simulink model "LUPA"  (R2025b)
settings: Solver=FixedStepAuto  StartTime=0.0  StopTime=inf  FixedStep=Ts  RelTol=1e-3
PreLoadFcn:
  | addpath(genpath('utils'))
model workspace (MAT data in the model file):
  Sig = Simulink.Signal
  Sig.Dimensions = -1
  Sig.DimensionsMode = 'auto'
  Sig.Complexity = 'auto'
  Sig.SampleTime = -1
  Sig.SamplingMode = 'auto'
  Sig.DataType = 'auto'
values from neighbouring files (symbols this model uses):
  C = 258.803991051052    (= 258.803991051)    [AOE_constants.m]
  CL = 13    [initLUPA.m]
  ExcelGains = table2array(ExcelGains)    [initLUPA.m]
  gainTstep = wavePeriod*10    (= 22.5)    [initLUPA.m]
  Kt = 7.86    [initLUPA.m]
  rampTime = 20    [initLUPA.m]
  sprocketPitchRadius = 0.101854    [initLUPA.m]
  Ts = 0.001    [initLUPA.m]
undefined symbols (not defined in the file or in its folder): AOE, DiscIntNeverNeededParam, drawWire_m, drawWire_mpers, eCATstate, linearPower_W, netForce_N, opState, pos_filt_rad, tet, vel_filt_radpers
libraries: slrealtimeethercatlib x16, slrealtimeloglib x10, simulink x7, dspfdesign x6, eeGeneralControl x3, slrealtimeutilitieslib x2, dspstat3 x2, slrealtimeptplib x1, slrealtimetgmanagement x1
(part 1 of 2)
settings Model: SimulationMode=external  ExtModeEnableFloating=off  Creator=HWRL user  LastModifiedBy=Wave User
settings SolverCC: ConcurrentTasks=on  PositivePriorityOrder=on
settings DataIOCC: ExternalInput=ds  LoadExternalInput=on
settings OptimizationCC: BlockReduction=off  OptimizeBlockIOStorage=off  ReuseModelBlockBuffer=off
settings DebuggingCC: TasksWithSamePriorityMsg=none  ParameterOverflowMsg=warning  ParameterPrecisionLossMsg=none  UnconnectedInputMsg=warning  UnconnectedOutputMsg=warning  UnconnectedLineMsg=warning
settings HardwareCC: ProdBitPerLong=64.0  ProdLongLongMode=on  ProdHWDeviceType=Intel->x86-64 (Linux 64)
settings ModelReferenceCC: EnableRefExpFcnMdlSchedulingChecks=on
settings SFSimCC: SimTargetLang=C++  SimDLTargetLibrary=mkl-dnn
settings RTWCC: SystemTargetFile=speedgoat.tlc  TemplateMakefile=slrealtime_default_tmf  RTWVerbose=off  Toolchain=Simulink Real-Time Toolchain  BuildConfiguration=Faster Runs  CodeExecutionProfiling=on  TargetLang=C++  GPUComputeCapability=3.5  DLArmComputeVersion=19.05  Description=Speedgoat Real-Time Target Machine
settings SimulinkRealTimeTargetCC: SLRTFileLogMaxRuns=1.0  ExtModeMaxTrigDuration=10.0  ExtModeStaticAllocSize=1000000.0  ExtModeTransport=0.0  MultiwordLength=2048.0  DynamicStringBufferSize=256.0  PreserveMATLABNamespacesInGeneratedCode=on  SubcomponentCodeInterfacePackaging=Reusable function  InstructionSetFMA=off  LogToMDFFile=off

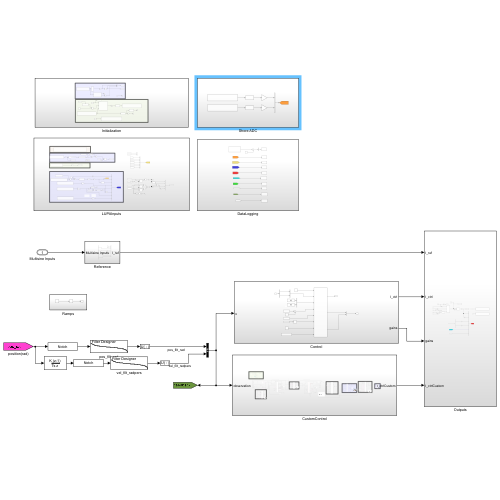
[thumbnail: Simulink's stored preview of the top-level diagram]
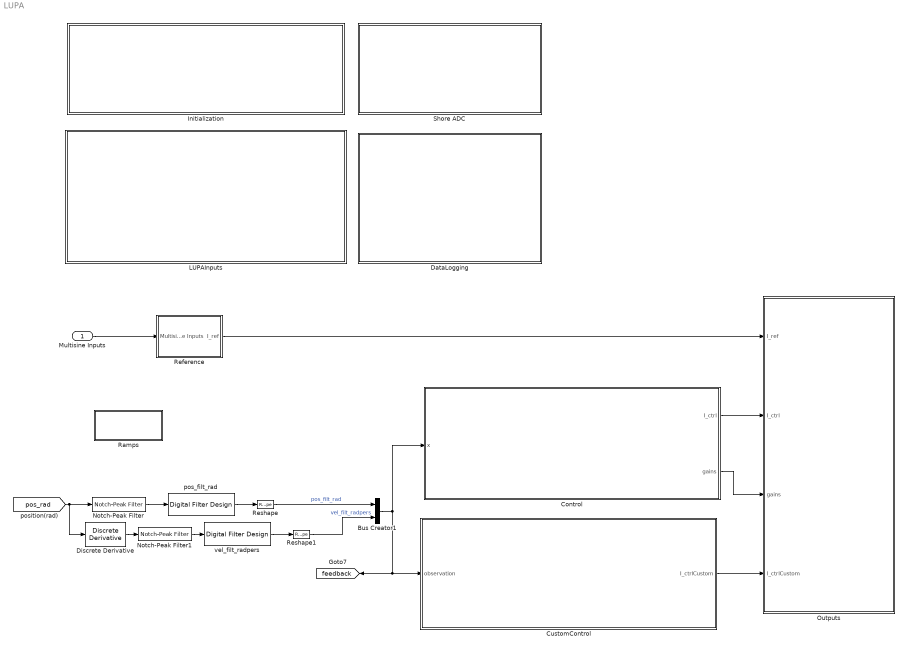
== system LUPA ==
  Multisine Inputs : Inport  OutDataTypeStr=Bus: refSigs
  Bus Creator1 : BusCreator  Inputs=pos_filt_rad,vel_filt_radpers
  Control : Subsystem
  CustomControl : Subsystem
  DataLogging : Subsystem
  Discrete Derivative : simulink/Discrete/Discrete Derivative  gainval=1.0  ICPrevScaledInput=0.0  OutMin=[]  OutMax=[]  OutDataType=fixdt(1, 16)  OutScaling=2^-10  DoSatur=off
  Initialization : Subsystem
  LUPAInputs : Subsystem
  Notch-Peak Filter : dspfdesign/Notch-Peak Filter  Specification=Bandwidth and center frequency  BandwidthPort=off  Bandwidth=10  QualityFactorPort=off  QualityFactor=5  CenterFrequencyPort=off  CenterFrequency=50  BandwidthCoefficientPort=off  BandwidthCoefficient=0.72654  CenterFrequencyCoefficientPort=off  CenterFrequencyCoefficient=0  Output=Notch  SampleRateMode=Specify on dialog  SampleRate=1000  SimulateUsing=Code generation
  Notch-Peak Filter1 : dspfdesign/Notch-Peak Filter  Specification=Bandwidth and center frequency  BandwidthPort=off  Bandwidth=10  QualityFactorPort=off  QualityFactor=5  CenterFrequencyPort=off  CenterFrequency=50  BandwidthCoefficientPort=off  BandwidthCoefficient=0.72654  CenterFrequencyCoefficientPort=off  CenterFrequencyCoefficient=0  Output=Notch  SampleRateMode=Specify on dialog  SampleRate=1000  SimulateUsing=Code generation
  Outputs : Subsystem
  Ramps : Subsystem
  Reference : Subsystem
  Reshape : Reshape
  Reshape1 : Reshape
  Shore ADC : Subsystem
  pos_filt_rad : dspfdesign/Digital Filter Design  mwdsp_browser_bugfix_var=off
  vel_filt_radpers : dspfdesign/Digital Filter Design  mwdsp_browser_bugfix_var=off
  tag scope: feedback=global
  wires:
  Control/1(I_ctrl) -> Outputs/2(I_ctrl)
  Bus Creator1/1 -> Control/1(x), CustomControl/1(observation), [feedback]
  [pos_rad] -> Discrete Derivative/1, Notch-Peak Filter/1
  Control/2(gains) -> Outputs/3(gains)
  CustomControl/1(I_ctrlCustom) -> Outputs/4(I_ctrlCustom)
  Reference/1(I_ref) -> Outputs/1(I_ref)
  Multisine Inputs/1 -> Reference/1(Multisine Inputs)
  Notch-Peak Filter/1 -> pos_filt_rad/1
  Notch-Peak Filter1/1 -> vel_filt_radpers/1
  Discrete Derivative/1 -> Notch-Peak Filter1/1
  pos_filt_rad/1 -> Reshape/1
  vel_filt_radpers/1 -> Reshape1/1
  Reshape/1 -> Bus Creator1/1  "pos_filt_rad"
  Reshape1/1 -> Bus Creator1/2  "vel_filt_radpers"

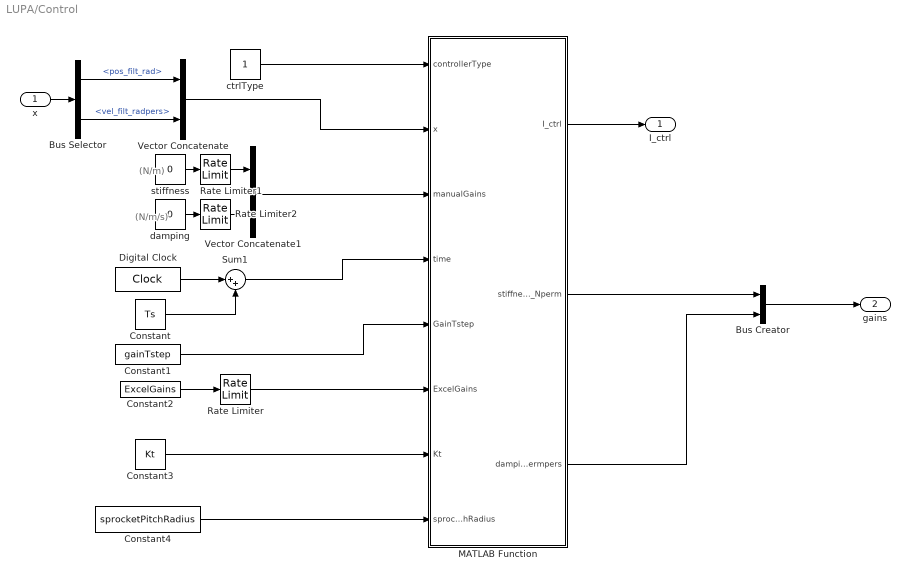
== system LUPA/Control ==
  note: (N/m/s)
  note: (N/m)
  x : Inport
  Bus Creator : BusCreator  Inputs=2
  Bus Selector : BusSelector  OutputSignals=pos_filt_rad,vel_filt_radpers
  Constant : Constant  Value=Ts
  Constant1 : Constant  Value=gainTstep
  Constant2 : Constant  Value=ExcelGains  VectorParams1D=off
  Constant3 : Constant  Value=Kt
  Constant4 : Constant  Value=sprocketPitchRadius
  Digital Clock : DigitalClock  SampleTime=Ts
  MATLAB Function : MATLAB Function  TreatAsAtomicUnit=on
  Rate Limiter : RateLimiter  RisingSlewLimit=200  FallingSlewLimit=-200  SampleTimeMode=inherited
  Rate Limiter1 : RateLimiter  RisingSlewLimit=200  FallingSlewLimit=-200  SampleTimeMode=inherited
  Rate Limiter2 : RateLimiter  RisingSlewLimit=200  FallingSlewLimit=-200  SampleTimeMode=inherited
  Sum1 : Sum  Inputs=|++
  Vector Concatenate : Concatenate  Mode=Multidimensional array
  Vector Concatenate1 : Concatenate  Mode=Multidimensional array
  ctrlType : Constant
  damping : Constant  Value=0
  stiffness : Constant  Value=0
  I_ctrl : Outport
  gains : Outport  Port=2
  wires:
  stiffness/1 -> Rate Limiter1/1
  Constant1/1 -> MATLAB Function/5(GainTstep)
  Constant/1 -> Sum1/2
  Vector Concatenate1/1 -> MATLAB Function/3(manualGains)
  Digital Clock/1 -> Sum1/1
  x/1 -> Bus Selector/1
  Sum1/1 -> MATLAB Function/4(time)
  Constant4/1 -> MATLAB Function/8(sprocketPitchRadius)
  damping/1 -> Rate Limiter2/1
  Vector Concatenate/1 -> MATLAB Function/2(x)
  ctrlType/1 -> MATLAB Function/1(controllerType)
  Constant3/1 -> MATLAB Function/7(Kt)
  Constant2/1 -> Rate Limiter/1
  Bus Selector/1 -> Vector Concatenate/1  "<pos_filt_rad>"
  Bus Selector/2 -> Vector Concatenate/2  "<vel_filt_radpers>"
  MATLAB Function/1(I_ctrl) -> I_ctrl/1
  MATLAB Function/2(stiffness_Nperm) -> Bus Creator/1
  MATLAB Function/3(damping_Npermpers) -> Bus Creator/2
  Bus Creator/1 -> gains/1
  Rate Limiter/1 -> MATLAB Function/6(ExcelGains)
  Rate Limiter1/1 -> Vector Concatenate1/1
  Rate Limiter2/1 -> Vector Concatenate1/2

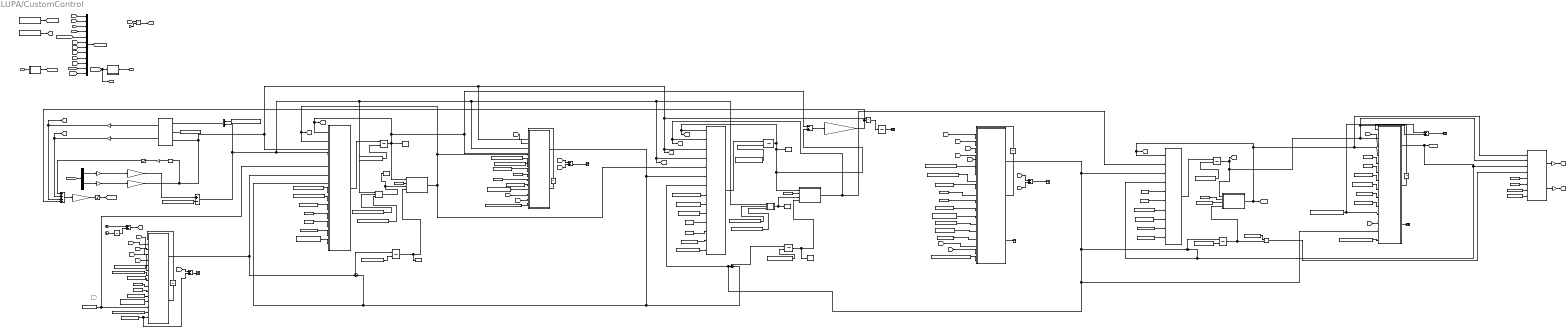
== system LUPA/CustomControl ==
  note: HWRL Code
  note: Outlet Piston Chamber 1 Valve
  note: Useful Power
  note: Outlet Tank Valve
  note: Outlet Piston Valve
  note: Inlet Piston valve
  observation : Inport
  Add1 : Sum  Inputs=+-
  Add{2..3,7,9} (4 alike) : Sum  Inputs=-+
  Add8 : Sum  Inputs=++++  RndMeth=Simplest
  Assertion : Assertion  AssertionFailFcn=Ch1C1 mass is zero
  Assertion1 : Assertion  AssertionFailFcn=Ch1C1 pressure is zero
  Assertion2 : Assertion  AssertionFailFcn=Ch2C1 pressure is zero  StopWhenAssertionFail=off
  Assertion3 : Assertion  AssertionFailFcn=Ch2C1 mass is zero  StopWhenAssertionFail=off
  Assertion4 : Assertion  AssertionFailFcn=Ch1C1 volume is zero
  Assertion5 : Assertion  AssertionFailFcn=Ch2C1 volume is zero  StopWhenAssertionFail=off
  Atmospheric pressure2 : Constant  Value=AOE.AtmPressure
  Atmospheric temperature : Constant  Value=AOE.AtmTemperature
  Bus Selector1 : BusSelector  OutputSignals=pos_filt_m,vel_filt_mpers
  Clock : Clock
  Clock1 : Clock
  Constant : Constant  Value=sprocketPitchRadius
  Constant1 : Constant  Value=Kt
  Constant{4..6,10,22,27,30,35,39,43,61} (11 alike) : Constant  Value=AOE.Rs
  Constant11 : Constant  Value=AOE.Cp
  Constant12 : Constant  Value=AOE.Chamber1.InitialAirMass
  Constant{2,14,24,37,56} (5 alike) : Constant  Value=AOE.Cylinder.HeatConvection
  Constant16 : Constant  Value=AOE.Chamber2.InitialPistonPosition
  Constant17 : Constant  Value=AOE.Cylinder.Diameter
  Constant18 : Constant  Value=AOE.Chamber2.InitialAirMass
  Constant19 : Constant  Value=AOE.Chamber1.InitialPressure
  Constant20 : Constant  Value=AOE.Chamber2.InitialPressure
  Constant21 : Constant  Value=AOE.OutletTankOrifice.CrossSectionalArea
  Constant{7,23,28,31,40,47,62} (7 alike) : Constant  Value=AOE.gma
  Constant25 : Constant  Value=AOE.Tank.InitialAirMass
  Constant{9,26,38,42,52,57,64} (7 alike) : Constant  Value=AOE.WaterTemperature
  Constant{8,29,41,46,49,51,63} (7 alike) : Constant  Value=AOE.Cylinder.CrossSectionalArea
  Constant{3,48,50,55,60} (5 alike) : Constant  Value=AOE.Tank.Volume
  Constant32 : Constant  Value=AOE.Tank.HeatConvection
  Constant33 : Constant  Value=AOE.Tank.InitialPressure
  Constant34 : Constant  Value=AOE.Tank.SurfaceArea
  Constant44 : Constant  Value=AOE.Chamber2.InitialPistonPosition
  Constant53 : Constant  Value=AOE.Tank.HeatConvection
  Constant54 : Constant  Value=AOE.Tank.SurfaceArea
  Constant58 : Constant  Value=AOE.Tank.HeatConvection
  Constant59 : Constant  Value=AOE.Tank.SurfaceArea
  Constant65 : Constant  Value=AOE.InletCylinderOrifice.CrossSectionalArea
  Constant66 : Constant  Value=AOE.OutletCylinderOrifice.CrossSectionalArea
  Constant67 : Constant  Value=AOE.Chamber1Chamber2Orifice.CrossSectionalArea
  Coulomb & Viscous Friction Unit1 : simulink/Discontinuities/Coulomb & Viscous Friction  offset=0  gain=AOE.Cylinder.CoulombFrictionGain
  CustomControl : BusCreator  Inputs=12
  Cyl D{,1..3} (4 alike) : Constant  Value=AOE.Cylinder.Diameter
  Determining Useful Energy : MATLAB Function
      settings: MinAlgLoopOccurrences=on
  Discrete-Time Integrator : DiscreteIntegrator  InitialConditionSource=external  InitialCondition=101.3  SampleTime=-1  LimitOutput=on  LowerSaturationLimit=0  ICPrevOutput=DiscIntNeverNeededParam  ICPrevScaledInput=DiscIntNeverNeededParam
  Discrete-Time Integrator10 : DiscreteIntegrator  InitialConditionSource=external  InitialCondition=1.2754*(10)*.25*pi*0.5^2  SampleTime=-1  LimitOutput=on  LowerSaturationLimit=0  ICPrevOutput=DiscIntNeverNeededParam  ICPrevScaledInput=DiscIntNeverNeededParam
  Discrete-Time Integrator11 : DiscreteIntegrator  InitialConditionSource=external  InitialCondition=1.2754*(2+.05)*.25*pi*2.14^2  SampleTime=-1  LimitOutput=on  LowerSaturationLimit=0  ICPrevOutput=DiscIntNeverNeededParam  ICPrevScaledInput=DiscIntNeverNeededParam
  Discrete-Time Integrator12 : DiscreteIntegrator  InitialConditionSource=external  InitialCondition=101.3  SampleTime=-1  LimitOutput=on  LowerSaturationLimit=0  ICPrevOutput=DiscIntNeverNeededParam  ICPrevScaledInput=DiscIntNeverNeededParam
  Discrete-Time Integrator2 : DiscreteIntegrator  InitialConditionSource=external  InitialCondition=1.2754*(2+.05)*.25*pi*2.14^2  SampleTime=-1  LimitOutput=on  LowerSaturationLimit=0  ICPrevOutput=DiscIntNeverNeededParam  ICPrevScaledInput=DiscIntNeverNeededParam
  Endstop Forces Unit1 : Subsystem
  Energy : DiscreteIntegrator  SampleTime=-1  LimitOutput=on  ICPrevOutput=DiscIntNeverNeededParam  ICPrevScaledInput=DiscIntNeverNeededParam
  Exergy : Gain
  Fh : Gain  OutDataTypeStr=double
  Fl : Gain  OutDataTypeStr=double
  Force : Gain  Gain=AOE.lambda^-3
  Force Limit : Saturate  UpperLimit=500  LowerLimit=-500
  ForceToCurrent : Subsystem
  From1 : From  Commented=on  GotoTag=TC1
  Gain : Gain  Gain=-1
  Gain1 : Gain  Gain=AOE.Cylinder.CrossSectionalArea
  Gain2 : Gain  Gain=AOE.lambda
  Gain3 : Gain  Gain=AOE.lambda^0.5
  P_pto : Product
  Power : Gain
  Pressure Chamber1 Box Unit1 : MATLAB Function
      settings: MinAlgLoopOccurrences=on
  Pressure Chamber2 Box Unit1 : MATLAB Function
  Pressure Tank Box Unit1 : MATLAB Function
      settings: MinAlgLoopOccurrences=on
  Pressure into Chamber 1 : Constant  Value=AOE.Chamber1.PressureIn
  Product2 : Product
  Product3 : Product  Inputs=/*
  Revised Cylinder Outlet Valve Model : MATLAB Function
      settings: MinAlgLoopOccurrences=on
  Revised Valve Model Chamber1Chamber2 Unit1 : MATLAB Function
      settings: MinAlgLoopOccurrences=on
  Revised Valve Model Inlet Unit1 : MATLAB Function
      settings: MinAlgLoopOccurrences=on
  Revised Valve Tank Outlet : MATLAB Function
      settings: MinAlgLoopOccurrences=on
  RotaryToLinear : Subsystem
  Saturation : Saturate  UpperLimit=AOE.Cylinder.CoulombFrictionLimit  LowerLimit=-AOE.Cylinder.CoulombFrictionLimit
  Sum : Sum  Inputs=+-
  Sum1 : Sum  Inputs=-+
  Sum2 : Sum  Inputs=-+
  Sum3 : Sum  Inputs=+|-
  Sum6 : Sum
  Temperature Chamber1 Box Unit1 : MATLAB Function
      settings: MinAlgLoopOccurrences=on
  Temperature Chamber2 Box Unit1 : MATLAB Function
      settings: MinAlgLoopOccurrences=on
  Temperature Tank Box Unit1 : MATLAB Function
  Terminator{,1..3,5..7} (7 alike) : Terminator
  Unit Delay{,1..4} (5 alike) : UnitDelay  SampleTime=-1
  Volume Chamber1 Box Unit1 : MATLAB Function
      settings: MinAlgLoopOccurrences=on
  Volume Chamber2 Box Unit1 : MATLAB Function
      settings: MinAlgLoopOccurrences=on
  cylinder equilibrium offset position{1,3..5} (4 alike) : Constant  Value=AOE.Chamber1.InitialPistonPosition
  cylinder equilibrium offset position2 : Constant  Value=AOE.Chamber2.InitialPistonPosition
  cylinder equilibrium offset position6 : Constant  Value=AOE.Chamber2.InitialPistonPosition
  cylinder initial offset : Constant  Value=AOE.Cylinder.InitialOffset
  cylinder total Length : Constant  Value=AOE.Cylinder.Length
  override2 : Constant  Value=AOE.OutletTankOrifice.CrackPressure
  pos_m : Gain
  tankPressure : DiscreteIntegrator  InitialConditionSource=external  InitialCondition=101.3  SampleTime=-1  LimitOutput=on  LowerSaturationLimit=0  ICPrevOutput=DiscIntNeverNeededParam  ICPrevScaledInput=DiscIntNeverNeededParam
  tempAmb2 : Constant  Value=AOE.AtmTemperature
  vel_mpers : Gain
  z_off : Sum  Inputs=+-  RndMeth=Simplest
  I_ctrlCustom : Outport
  tag scope: CustomControl=global, Kt=global, P_PTO=global, sprocketPitchRadius=global
  wires:
  Constant/1 -> [sprocketPitchRadius]
  Constant1/1 -> [Kt]
  ForceToCurrent/1(Out1) -> I_ctrlCustom/1
  [F_PTO] -> P_pto/1
  [v] -> P_pto/2
  P_pto/1 -> [P_PTO]  "P_PTO"
  observation/1 -> RotaryToLinear/1(rotational)
  CustomControl/1 -> [CustomControl]
  [F_PTO] -> CustomControl/1  "F_PTO"
  [z] -> CustomControl/2  "z"
  [v] -> CustomControl/3  "v"
  [P_PTO] -> CustomControl/4  "P_PTO"
  [EnableCustControl] -> CustomControl/5  "customControlEnable"
  Clock/1 -> Add1/1
  Volume Chamber2 Box Unit1/1(V) -> Assertion5/1, Temperature Chamber2 Box Unit1/3(V)  "Chamber2 volume"
  Revised Cylinder Outlet Valve Model/2(mdotMax) -> Unit Delay2/1
  Constant2/1 -> Revised Valve Model Chamber1Chamber2 Unit1/13(hC)
  Pressure into Chamber 1/1 -> Add9/2, Revised Valve Model Inlet Unit1/16(Pin)
  Endstop Forces Unit1/1(F_stop_hi) -> Fl/1  "Fstop_high"
  Atmospheric pressure2/1 -> Determining Useful Energy/8(Pamb)
  Discrete-Time Integrator11/1 -> Temperature Chamber1 Box Unit1/4(m), Assertion/1  "chamber1 air mass"
  Volume Chamber1 Box Unit1/1(V) -> Assertion4/1, Temperature Chamber1 Box Unit1/3(V)  "Chamber1 Volume"
  [response] -> Bus Selector1/1
  Cyl D3/1 -> Revised Valve Model Chamber1Chamber2 Unit1/9(DC)
  [PC1] -> Add9/1
  cylinder equilibrium offset position6/1 -> Revised Cylinder Outlet Valve Model/7(LC)
  tankPressure/1 -> [PT], Temperature Tank Box Unit1/1(P), Revised Valve Tank Outlet/3(PT), Determining Useful Energy/2(P), Add3/2  "Tank pressure"
  Unit Delay4/1 -> Revised Valve Model Inlet Unit1/1(mdotMaxOld)
  Constant56/1 -> Revised Valve Model Inlet Unit1/13(hC)
  Constant28/1 -> Pressure Chamber2 Box Unit1/12(gma)
  Constant32/1 -> Pressure Tank Box Unit1/7(h)
  [xDot] -> Revised Valve Model Inlet Unit1/5(xdot)
  override2/1 -> Add3/1, Revised Valve Tank Outlet/11(Pcrack)
  [TC1] -> Revised Valve Model Inlet Unit1/4(TC1)
  Constant4/1 -> Temperature Chamber1 Box Unit1/2(Rs)
  [TimeStep] -> Revised Cylinder Outlet Valve Model/2(TimeStep)
  Unit Delay1/1 -> Add1/2
  Constant39/1 -> Revised Valve Model Chamber1Chamber2 Unit1/10(Rs)
  [PC1] -> Add7/2
  Constant8/1 -> Pressure Chamber1 Box Unit1/9(A)
  Sum2/1 -> Discrete-Time Integrator2/1
  Constant57/1 -> Revised Valve Tank Outlet/7(Tw)
  Revised Valve Tank Outlet/3(beta) -> Terminator5/1
  Discrete-Time Integrator10/1 -> Product3/2, Temperature Tank Box Unit1/4(m)  "Tank air mas"
  Constant60/1 -> Revised Valve Tank Outlet/9(VT)
  Constant35/1 -> Temperature Tank Box Unit1/2(Rs)
  Gain1/1 -> Add8/4, Product2/2  "Pressure Potential Force"
  [TC2] -> Revised Valve Model Chamber1Chamber2 Unit1/15(TC2)
  Cyl D1/1 -> Revised Cylinder Outlet Valve Model/9(DC)
  Constant61/1 -> Revised Valve Model Inlet Unit1/10(Rs)
  Product3/1 -> Determining Useful Energy/4(Density)
  Constant12/1 -> Discrete-Time Integrator11/2
  Constant66/1 -> Revised Cylinder Outlet Valve Model/19(A)
  Unit Delay2/1 -> Revised Cylinder Outlet Valve Model/1(mdotMaxOld)
  Revised Cylinder Outlet Valve Model/1(MassFlow) -> Revised Valve Tank Outlet/13(mDotIn), Pressure Chamber2 Box Unit1/7(mdot3), Sum2/1, Sum3/1, Pressure Tank Box Unit1/3(mdot1)  "Outlet cylinder"
  cylinder equilibrium offset position3/1 -> Revised Valve Model Chamber1Chamber2 Unit1/7(LC)
  Constant64/1 -> Revised Valve Model Inlet Unit1/12(Tw)
  Add8/1 -> Force/1  "Total Reaction Force"
  Constant27/1 -> Pressure Chamber2 Box Unit1/11(Rs)
  [TC2] -> Revised Valve Tank Outlet/12(TC)
  [TC2] -> Revised Cylinder Outlet Valve Model/4(TC)
  Constant6/1 -> Pressure Chamber1 Box Unit1/11(Rs)
  Constant62/1 -> Revised Valve Model Inlet Unit1/11(gma)
  Constant53/1 -> Revised Cylinder Outlet Valve Model/14(hT)
  Constant26/1 -> Pressure Chamber2 Box Unit1/13(Tw)
  Add1/1 -> [TimeStep]
  [PT] -> Revised Cylinder Outlet Valve Model/17(PT)
  Discrete-Time Integrator2/1 -> Temperature Chamber2 Box Unit1/4(m), Assertion3/1  "Chamber2 air mass"
  [TimeStep] -> Revised Valve Tank Outlet/2(TimeStep)
  Add2/1 -> Terminator2/1
  Coulomb & Viscous Friction Unit1/1 -> Gain/1
  Revised Valve Model Chamber1Chamber2 Unit1/2(mdotMax) -> Unit Delay3/1
  Unit Delay/1 -> Revised Valve Tank Outlet/1(mdotMaxOld)
  cylinder equilibrium offset position5/1 -> Revised Valve Model Inlet Unit1/7(LC)
  Sum6/1 -> Endstop Forces Unit1/1(x)  "Piston Position"
  Constant21/1 -> Revised Valve Tank Outlet/14(A)
  Constant44/1 -> Sum6/1
  Constant43/1 -> Revised Cylinder Outlet Valve Model/10(Rs)
  Pressure Chamber1 Box Unit1/1(Pdot) -> Discrete-Time Integrator/1  "pdot(t)"
  Gain2/1 -> z_off/1  "x"
  Constant63/1 -> Revised Valve Model Inlet Unit1/8(AC)
  Constant48/1 -> Temperature Tank Box Unit1/3(V)
  Add7/1 -> Terminator6/1
  Endstop Forces Unit1/2(F_stop_lo) -> Fh/1  "Fstop_high"
  Cyl D2/1 -> Revised Valve Model Inlet Unit1/9(DC)
  Gain3/1 -> Coulomb & Viscous Friction Unit1/1, Pressure Chamber1 Box Unit1/3(xdot), Revised Valve Model Chamber1Chamber2 Unit1/3(xdot), [xDot], Pressure Chamber2 Box Unit1/3(xdot), Product2/1, Endstop Forces Unit1/3(xdot(t))  "Xdot"
  Revised Valve Model Inlet Unit1/1(MassFlow) -> Sum/1, Pressure Chamber1 Box Unit1/6(mdot1)  "Inlet Cylinder MassFlow to Cyl"
  Constant17/1 -> Pressure Chamber2 Box Unit1/10(D)
  Constant58/1 -> Revised Valve Tank Outlet/8(hT)
  Constant65/1 -> Revised Valve Model Inlet Unit1/15(A)
  Determining Useful Energy/1(Exergy) -> Exergy/1
  Revised Cylinder Outlet Valve Model/3(beta) -> Terminator1/1
  Constant37/1 -> Pressure Chamber1 Box Unit1/14(h)
  Constant7/1 -> Pressure Chamber1 Box Unit1/12(gma)
  [TimeStep] -> Revised Valve Model Chamber1Chamber2 Unit1/2(TimeStep)
  Discrete-Time Integrator/1 -> Pressure Chamber1 Box Unit1/1(P), [PC1], Revised Valve Model Chamber1Chamber2 Unit1/5(PC1), Sum1/1, Assertion1/1, Temperature Chamber1 Box Unit1/1(P)  "Chamber1 Pressure"
  cylinder equilibrium offset position4/1 -> Pressure Chamber1 Box Unit1/8(L)
  Constant40/1 -> Revised Valve Model Chamber1Chamber2 Unit1/11(gma)
  Constant9/1 -> Pressure Chamber1 Box Unit1/13(Tw)
  Constant14/1 -> Revised Cylinder Outlet Valve Model/13(hC)
  cylinder equilibrium offset position1/1 -> Volume Chamber1 Box Unit1/3(L)
  Revised Valve Tank Outlet/2(mdotMax) -> Unit Delay/1
  [PC1] -> Revised Valve Model Inlet Unit1/3(PC1)
  Temperature Tank Box Unit1/1(T) -> [Temp], Determining Useful Energy/1(T), Revised Valve Tank Outlet/4(TT), Pressure Tank Box Unit1/1(T), [TT]  "Unit1 Tank temp"
  Constant49/1 -> Volume Chamber2 Box Unit1/2(A)
  Constant55/1 -> Revised Cylinder Outlet Valve Model/16(VT)
  Gain/1 -> Saturation/1
  Constant22/1 -> Revised Valve Tank Outlet/5(Rs)
  Clock1/1 -> Unit Delay1/1
  Discrete-Time Integrator12/1 -> Pressure Chamber2 Box Unit1/1(P), [PC2], Assertion2/1, Temperature Chamber2 Box Unit1/1(P), Sum1/2  "Chamber2 Pressure"
  Revised Valve Model Chamber1Chamber2 Unit1/1(MassFlow) -> Sum2/2, Pressure Chamber1 Box Unit1/7(mdot3), Sum/2, Pressure Chamber2 Box Unit1/6(mdot1)  "mdot(t)"
  tempAmb2/1 -> Determining Useful Energy/7(Tamb)
  [xDot] -> Revised Cylinder Outlet Valve Model/5(xdot)
  [PT] -> Add2/1
  Constant24/1 -> Pressure Chamber2 Box Unit1/14(h)
  Product2/1 -> Energy/1
  [PC2] -> Revised Valve Model Chamber1Chamber2 Unit1/14(PC2)
  cylinder total Length/1 -> Endstop Forces Unit1/2(Total length)
  Constant11/1 -> Determining Useful Energy/5(Cp)
  Saturation/1 -> Add8/1  "Motion Friction"
  [PC2] -> Add7/1
  Constant41/1 -> Revised Valve Model Chamber1Chamber2 Unit1/8(AC)
  Add3/1 -> Terminator3/1
  Constant3/1 -> Product3/1
  Constant19/1 -> Discrete-Time Integrator/2
  Determining Useful Energy/2(Power) -> Power/1
  Constant31/1 -> Pressure Tank Box Unit1/6(gma)
  Sum3/1 -> Discrete-Time Integrator10/1  "mdot1-mdot2"
  Constant34/1 -> Pressure Tank Box Unit1/8(a)
  [x] -> Revised Valve Model Inlet Unit1/6(x)
  Sum/1 -> Discrete-Time Integrator11/1  "mdot1-mdot2"
  [PC2] -> Revised Cylinder Outlet Valve Model/3(PC)
  Constant54/1 -> Revised Cylinder Outlet Valve Model/15(aT)
  cylinder equilibrium offset position2/1 -> Volume Chamber2 Box Unit1/3(L)
  Unit Delay3/1 -> Revised Valve Model Chamber1Chamber2 Unit1/1(mdotMaxOld)
  Constant30/1 -> Pressure Tank Box Unit1/5(Rs)
  Constant25/1 -> Discrete-Time Integrator10/2
  Constant33/1 -> tankPressure/2
  Constant51/1 -> Revised Cylinder Outlet Valve Model/8(AC)
  Cyl D/1 -> Pressure Chamber1 Box Unit1/10(D)
  Constant23/1 -> Revised Valve Tank Outlet/6(gma)
  Constant38/1 -> Pressure Tank Box Unit1/10(Tw)
  Constant20/1 -> Discrete-Time Integrator12/2
  [TimeStep] -> Revised Valve Model Inlet Unit1/2(TimeStep)
  Pressure Chamber2 Box Unit1/1(Pdot) -> Discrete-Time Integrator12/1  "pdot(t)"
  Revised Valve Model Inlet Unit1/2(mdotMax) -> Unit Delay4/1
  Constant47/1 -> Revised Cylinder Outlet Valve Model/11(gma)
  Constant46/1 -> Volume Chamber1 Box Unit1/2(A)
  Atmospheric temperature/1 -> Revised Valve Model Inlet Unit1/14(Tamb), Pressure Chamber1 Box Unit1/5(Tin1)
  Constant18/1 -> Discrete-Time Integrator2/2
  Constant59/1 -> Revised Valve Tank Outlet/10(aT)
  Sum1/1 -> Gain1/1
  [TT] -> Revised Cylinder Outlet Valve Model/18(TT)
  Constant52/1 -> Revised Cylinder Outlet Valve Model/12(Tw)
  Temperature Chamber1 Box Unit1/1(T) -> Pressure Chamber2 Box Unit1/5(Tin1), Pressure Chamber1 Box Unit1/2(T), [TC1], Revised Valve Model Chamber1Chamber2 Unit1/6(TC1)  "chamber1 temp"
  Constant42/1 -> Revised Valve Model Chamber1Chamber2 Unit1/12(Tw)
  Force/1 -> Force Limit/1
  Revised Valve Tank Outlet/1(MassFlow) -> [MassFlow], Sum3/2, Pressure Tank Box Unit1/4(mdot2), Determining Useful Energy/3(mDot)  "Unit1 Outlet tank mdot"
  Temperature Chamber2 Box Unit1/1(T) -> Pressure Chamber2 Box Unit1/2(T), [TC2], Pressure Tank Box Unit1/2(Tin)  "Chamber2 temperature"
  Constant10/1 -> Determining Useful Energy/6(Rs)
  Constant5/1 -> Temperature Chamber2 Box Unit1/2(Rs)
  [PC2] -> Add2/2
  z_off/1 -> Volume Chamber1 Box Unit1/1(x), Revised Valve Model Chamber1Chamber2 Unit1/4(x), Pressure Chamber2 Box Unit1/4(x), [x], Volume Chamber2 Box Unit1/1(x), Pressure Chamber1 Box Unit1/4(x), Sum6/2  "x"
  Energy/1 -> Terminator7/1
  [x] -> Revised Cylinder Outlet Valve Model/6(x)
  Pressure Tank Box Unit1/1(Pdot) -> tankPressure/1
  Constant50/1 -> Pressure Tank Box Unit1/9(V)
  Constant67/1 -> Revised Valve Model Chamber1Chamber2 Unit1/16(A)
  Constant16/1 -> Pressure Chamber2 Box Unit1/8(L)
  cylinder initial offset/1 -> z_off/2
  Add9/1 -> Terminator/1
  Constant29/1 -> Pressure Chamber2 Box Unit1/9(A)
  RotaryToLinear/1(linear) -> [response]
  [Force] -> [F_PTO], ForceToCurrent/1(Force_N)
  [Power] -> CustomControl/6  "Power"
  [Ex] -> CustomControl/7  "Ex"
  [Fl] -> CustomControl/8  "Fl"
  [Fh] -> CustomControl/9  "Fh"
  Bus Selector1/1 -> pos_m/1  "<pos_filt_m>"
  Bus Selector1/2 -> vel_mpers/1  "<vel_filt_mpers>"
  Fl/1 -> [Fl], Add8/3
  Fh/1 -> [Fh], Add8/2
  Exergy/1 -> [Ex]
  [PT] -> CustomControl/10  "PT"
  Power/1 -> [Power]
  [MassFlow] -> CustomControl/11  "MassFlow"
  [Temp] -> CustomControl/12
  pos_m/1 -> Gain2/1
  vel_mpers/1 -> Gain3/1
  Force Limit/1 -> [Force]

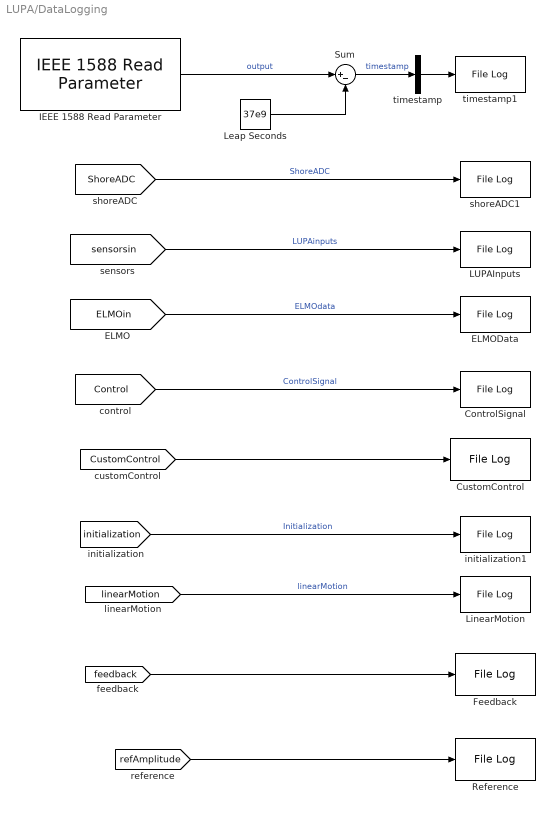
== system LUPA/DataLogging ==
  ControlSignal : slrealtimeloglib/File Log  decimation=decimationLog  inputProcessing=Elements as channels (sample based)
  CustomControl : slrealtimeloglib/File Log  decimation=decimationLog  inputProcessing=Elements as channels (sample based)
  ELMOData : slrealtimeloglib/File Log  decimation=decimationLog  inputProcessing=Elements as channels (sample based)
  Feedback : slrealtimeloglib/File Log  decimation=1  inputProcessing=Elements as channels (sample based)
  IEEE 1588 Read Parameter : slrealtimeptplib/IEEE 1588 Read Parameter  Priority=1  ID=1  param=1. System time (nanosecond)  sample_time=Ts
  LUPAInputs : slrealtimeloglib/File Log  decimation=decimationLog  inputProcessing=Elements as channels (sample based)
  Leap Seconds : Constant  Value=37e9  OutDataTypeStr=double
  LinearMotion : slrealtimeloglib/File Log  decimation=decimationLog  inputProcessing=Elements as channels (sample based)
  Reference : slrealtimeloglib/File Log  decimation=1  inputProcessing=Elements as channels (sample based)
  Sum : Sum  Inputs=|+-
  initialization1 : slrealtimeloglib/File Log  decimation=decimationLog  inputProcessing=Elements as channels (sample based)
  shoreADC1 : slrealtimeloglib/File Log  decimation=decimationLog  inputProcessing=Elements as channels (sample based)
  timestamp : BusCreator  Inputs=timestamp
  timestamp1 : slrealtimeloglib/File Log  decimation=decimationLog  inputProcessing=Elements as channels (sample based)
  wires:
  [ELMOin] -> ELMOData/1  "ELMOdata"
  [Control] -> ControlSignal/1  "ControlSignal"
  IEEE 1588 Read Parameter/1 -> Sum/1  "output"
  Sum/1 -> timestamp/1  "timestamp"
  timestamp/1 -> timestamp1/1
  Leap Seconds/1 -> Sum/2
  [initialization] -> initialization1/1  "Initialization"
  [sensorsin] -> LUPAInputs/1  "LUPAinputs"
  [ShoreADC] -> shoreADC1/1  "ShoreADC"
  [linearMotion] -> LinearMotion/1  "linearMotion"
  [feedback] -> Feedback/1
  [CustomControl] -> CustomControl/1
  [refAmplitude] -> Reference/1

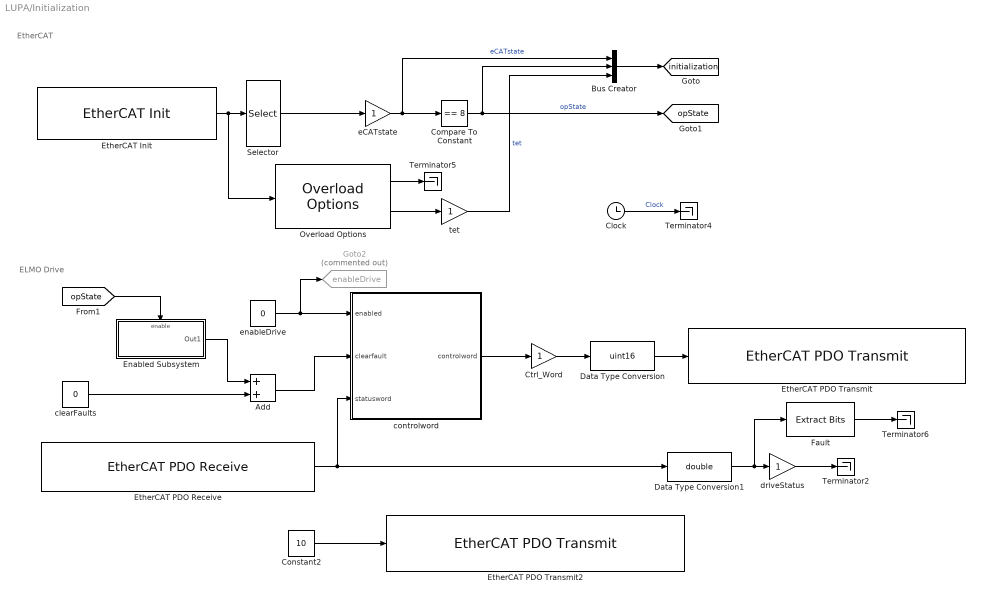
== system LUPA/Initialization ==
  note: ELMO Drive
  note: EtherCAT
  Add : Sum
  Bus Creator : BusCreator  Inputs=eCATstate,opState,tet
  Clock : Clock
  Compare To Constant : simulink/Logic and Bit Operations/Compare To Constant  relop===  const=8  OutDataTypeStr=boolean
  Constant2 : Constant  Value=10  OutDataTypeStr=int8
  Ctrl_Word : Gain
  Data Type Conversion : DataTypeConversion  OutDataTypeStr=uint16  SaturateOnIntegerOverflow=off  RndMeth=Floor
  Data Type Conversion1 : DataTypeConversion  OutDataTypeStr=double  SaturateOnIntegerOverflow=off  RndMeth=Floor
  Enabled Subsystem : Subsystem  TreatAsAtomicUnit=on
  EtherCAT Init : slrealtimeethercatlib/EtherCAT Init  Priority=0  config_file=C:\Software\LUPA\Simulink\EtherCAT\LUPAxml.xml  device_id=0  portnum=1  initstate=2  dctuning=0  enaDebug=0  logFile='c:\dbglog.txt'  sample_time=0.001000  DCMode=2
  EtherCAT PDO Receive : slrealtimeethercatlib/EtherCAT PDO Receive  Priority=2  sig_name=Drive 8 (Elmo Drive ).Inputs.Status word  sig_offset=1784  sig_type=uint16  type_size=16  sig_dim=1  device_id=0  sample_time=0.001000
  EtherCAT PDO Transmit : slrealtimeethercatlib/EtherCAT PDO Transmit  Priority=3  sig_name=Drive 8 (Elmo Drive ).Outputs.Control word  sig_offset=1784  sig_type=uint16  type_size=16  sig_dim=1  device_id=0  sample_time=0.001000
  EtherCAT PDO Transmit2 : slrealtimeethercatlib/EtherCAT PDO Transmit  Priority=3  sig_name=Drive 8 (Elmo Drive ).Outputs_1.Mode of operation  sig_offset=1800  sig_type=int8  type_size=8  sig_dim=1  device_id=0  sample_time=0.001000
  Fault : simulink/Logic and Bit Operations/Extract Bits  bitsToExtract=Range of bits  numBits=8  bitIdxRange=[3]  outScalingMode=Preserve fixed-point scaling
  Goto2 : Goto  Commented=on  GotoTag=enableDrive  TagVisibility=global
  Overload Options : slrealtimetgmanagement/Overload Options  startupDur=1  startupDurSrc=Tunable Parameter  maxOverload=0  maxOverloadSrc=Tunable Parameter  TETFlag=on
  Selector : Selector  InputPortWidth=6  IndexOptions=Index vector (dialog)  Indices=2  OutputSizes=1
  Terminator{2,4..6} (4 alike) : Terminator
  clearFaults : Constant  Value=0
  controlword : MATLAB Function  TreatAsAtomicUnit=on
  driveStatus : Gain
  eCATstate : Gain  OutDataTypeStr=double
  enableDrive : Constant  Value=0
  tet : Gain  OutDataTypeStr=double
  tag scope: initialization=global, opState=global
  wires:
  EtherCAT Init/1 -> Overload Options/1, Selector/1
  Selector/1 -> eCATstate/1
  Compare To Constant/1 -> [opState], Bus Creator/2  "opState"
  EtherCAT PDO Receive/1 -> Data Type Conversion1/1, controlword/3(statusword)
  Constant2/1 -> EtherCAT PDO Transmit2/1
  Data Type Conversion1/1 -> Fault/1, driveStatus/1
  controlword/1(controlword) -> Ctrl_Word/1
  Data Type Conversion/1 -> EtherCAT PDO Transmit/1
  driveStatus/1 -> Terminator2/1
  Ctrl_Word/1 -> Data Type Conversion/1
  enableDrive/1 -> Goto2/1, controlword/1(enabled)
  eCATstate/1 -> Bus Creator/1, Compare To Constant/1  "eCATstate"
  Clock/1 -> Terminator4/1  "Clock"
  Bus Creator/1 -> [initialization]
  Overload Options/2 -> tet/1
  tet/1 -> Bus Creator/3  "tet"
  Overload Options/1 -> Terminator5/1
  Fault/1 -> Terminator6/1
  Enabled Subsystem/1(Out1) -> Add/1
  [opState] -> Enabled Subsystem/Enable
  Add/1 -> controlword/2(clearfault)
  clearFaults/1 -> Add/2

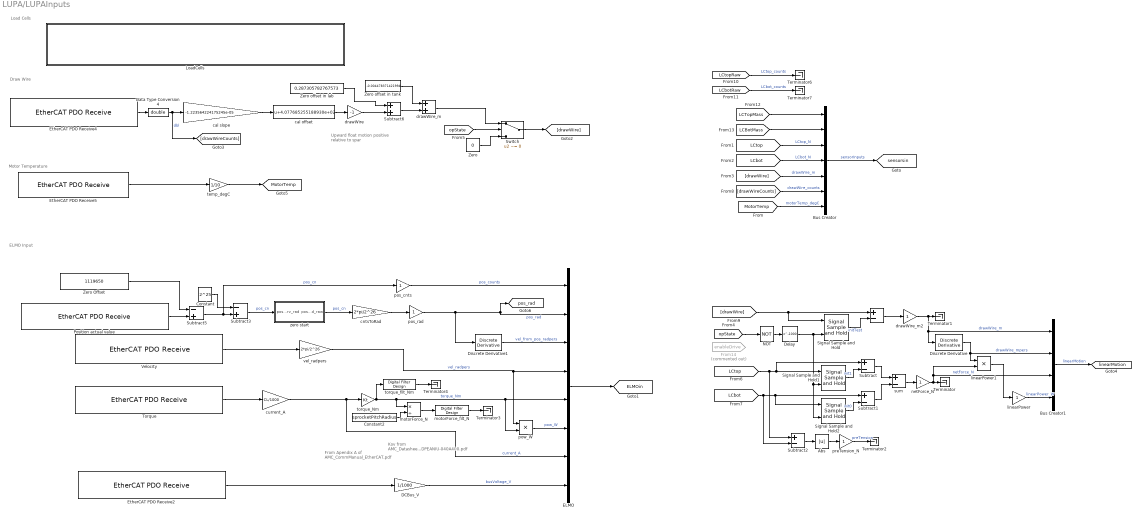
== system LUPA/LUPAInputs ==
  note: Load Cells
  note: Upward float motion
      | positive relative to spar
  note: Draw Wire
  note: Motor Temperature
  note: From Apendix A of AMC_CommManual_EtherCAT.pdf
  note: ELMO Input
  note: Kov from AMC_Datasheet_DPEANIU-040A400.pdf
  " " : Sum  Inputs=+-
  Abs : Abs  SaturateOnIntegerOverflow=off
  Bus Creator : BusCreator  Inputs=7
  Bus Creator1 : BusCreator  Inputs=drawWire_m,drawWire_mpers,netForce_N,linearPower_W
  Constant : Constant  Value=2^25
  Constant2 : Constant  Value=sprocketPitchRadius
  DCBus_V : Gain  Gain=1/1000  OutDataTypeStr=double
  Data Type Conversion4 : DataTypeConversion  OutDataTypeStr=double  SaturateOnIntegerOverflow=off  RndMeth=Floor
  Delay : Delay  DelayLength=1000
  Discrete Derivative : simulink/Discrete/Discrete Derivative  gainval=1.0  ICPrevScaledInput=0.0  OutMin=[]  OutMax=[]  OutDataType=fixdt(1, 16)  OutScaling=2^-10  DoSatur=off
  Discrete Derivative1 : simulink/Discrete/Discrete Derivative  gainval=1.0  ICPrevScaledInput=0.0  OutMin=[]  OutMax=[]  OutDataType=fixdt(1, 16)  OutScaling=2^-10  DoSatur=off
  ELMO : BusCreator  Inputs=8
  EtherCAT PDO Receive2 : slrealtimeethercatlib/EtherCAT PDO Receive  Priority=2  sig_name=Drive 8 (Elmo Drive ).Inputs_7.DC link circuit voltage  sig_offset=1960  sig_type=uint32  type_size=32  sig_dim=1  device_id=0  sample_time=0.001000
  EtherCAT PDO Receive4 : slrealtimeethercatlib/EtherCAT PDO Receive  Priority=2  sig_name=Term 4 (EL5002).SSI Inputs Channel 1.Counter value  sig_offset=712  sig_type=uint32  type_size=32  sig_dim=1  device_id=0  sample_time=0.001000
  EtherCAT PDO Receive5 : slrealtimeethercatlib/EtherCAT PDO Receive  Priority=2  sig_name=Term 7 (EL3202).RTD Inputs Channel 1.Value  sig_offset=1640  sig_type=int16  type_size=16  sig_dim=1  device_id=0  sample_time=0.001000
  From14 : From  Commented=on  GotoTag=enableDrive  TagVisibility=global
  LoadCells : Subsystem
  NOT : Logic  Operator=NOT  IconShape=distinctive  AllPortsSameDT=off  OutDataTypeStr=boolean
  Position actual value : slrealtimeethercatlib/EtherCAT PDO Receive  Priority=2  sig_name=Drive 8 (Elmo Drive ).Inputs_3.Actual position [counts]  sig_offset=1848  sig_type=int32  type_size=32  sig_dim=1  device_id=0  sample_time=0.001000
  Signal Sample and Hold : eeGeneralControl/Signal Sample and Hold  LabelModeActiveChoice=Discrete  x0=0  Ts=Ts
      settings: LibrarySourceBlock=ee_sl_lib/General Control/Signal Sample and Hold
  Signal Sample and Hold1 : eeGeneralControl/Signal Sample and Hold  LabelModeActiveChoice=Discrete  x0=0  Ts=Ts
      settings: LibrarySourceBlock=ee_sl_lib/General Control/Signal Sample and Hold
  Signal Sample and Hold2 : eeGeneralControl/Signal Sample and Hold  LabelModeActiveChoice=Discrete  x0=0  Ts=Ts
      settings: LibrarySourceBlock=ee_sl_lib/General Control/Signal Sample and Hold
  Subtract : Sum  Inputs=+-
  Subtract1 : Sum  Inputs=+-
  Subtract2 : Sum  Inputs=+-
  Subtract3 : Sum  Inputs=-+
  Subtract5 : Sum  Inputs=-+  OutDataTypeStr=double
  Subtract6 : Sum
  Switch : Switch  Criteria=u2 ~= 0  SaturateOnIntegerOverflow=off  InputSameDT=off
  Terminator{,1..4,6..7} (7 alike) : Terminator
  Torque : slrealtimeethercatlib/EtherCAT PDO Receive  Priority=2  sig_name=Drive 8 (Elmo Drive ).Inputs_9.Current actual value  sig_offset=2024  sig_type=int16  type_size=16  sig_dim=1  device_id=0  sample_time=0.001000
  Velocity : slrealtimeethercatlib/EtherCAT PDO Receive  Priority=2  sig_name=Drive 8 (Elmo Drive ).Inputs_5.Velocity sensor actual value [counts/sec]  sig_offset=1912  sig_type=int32  type_size=32  sig_dim=1  device_id=0  sample_time=0.001000
  Zero : Constant  Value=0  OutDataTypeStr=double
  Zero Offset : Constant  Value=1119650
  Zero offset in lab : Constant  Value=0.287305782767573
  Zero offset in tank : Constant  Value=-0.004478371421994
  cal offset : Bias  Bias=4.077685255188930e+02  SaturateOnIntegerOverflow=off
  cal slope : Gain  Gain=-1.223564224175245e-05
  cntsToRad : Gain  Gain=2*pi/2^26  OutDataTypeStr=double
  current_A : Gain  Gain=CL/1000  OutDataTypeStr=double
  drawWire : Gain  Gain=-1
  drawWire_m : Sum
  drawWire_m2 : Gain
  linearPower : Gain
  linearPower1 : Product
  motorForce_N : Product  Inputs=*/
  motorForce_filt_N : dspfdesign/Digital Filter Design  mwdsp_browser_bugfix_var=off
  netForce_N : Gain
  pos_cnts : Gain
  pos_rad : Gain
  pow_W : Product
  preTension_N : Gain
  sum : Sum  Inputs=+-
  temp_degC : Gain  Gain=1/10  OutDataTypeStr=double
  torque_Nm : Gain  Gain=Kt
  torque_filt_Nm : dspfdesign/Digital Filter Design  mwdsp_browser_bugfix_var=off
  vel_radpers : Gain  Gain=2*pi/2^26  OutDataTypeStr=double
  zero start : Subsystem
  tag scope: ELMOin=global, MotorTemp=global, linearMotion=global, pos_rad=global, sensorsin=global
  wires:
  [opState] -> Switch/2
  EtherCAT PDO Receive4/1 -> Data Type Conversion4/1
  Data Type Conversion4/1 -> [drawWireCounts], cal slope/1  "dbl"
  Zero/1 -> Switch/3
  temp_degC/1 -> [MotorTemp]
  EtherCAT PDO Receive5/1 -> temp_degC/1
  Bus Creator/1 -> [sensorsin]  "sensorInputs"
  [drawWire] -> Bus Creator/5  "drawWire_m"
  [LCtop] -> Bus Creator/3  "LCtop_N"
  [MotorTemp] -> Bus Creator/7  "motorTemp_degC"
  [LCbot] -> Bus Creator/4  "LCbot_N"
  torque_Nm/1 -> torque_filt_Nm/1, pow_W/2, ELMO/5, motorForce_N/1  "torque_Nm"
  Discrete Derivative1/1 -> ELMO/3  "vel_from_pos_radpers"
  EtherCAT PDO Receive2/1 -> DCBus_V/1
  vel_radpers/1 -> pow_W/1, ELMO/4  "vel_radpers"
  pos_rad/1 -> Discrete Derivative1/1, [pos_rad], ELMO/2  "pos_rad"
  Torque/1 -> current_A/1
  ELMO/1 -> [ELMOin]
  DCBus_V/1 -> ELMO/8  "busVoltage_V"
  Constant/1 -> Subtract3/1
  Subtract5/1 -> pos_cnts/1, Subtract3/2  "pos_cn"
  current_A/1 -> torque_Nm/1, ELMO/7  "current_A"
  pow_W/1 -> ELMO/6  "pow_W"
  cntsToRad/1 -> pos_rad/1
  [drawWire] -> Signal Sample and Hold/1, " "/1
  drawWire_m2/1 -> Bus Creator1/1, Discrete Derivative/1, Terminator1/1  "drawWire_m"
  netForce_N/1 -> Bus Creator1/3, linearPower1/2, Terminator/1  "netForce_N"
  sum/1 -> netForce_N/1
  Abs/1 -> preTension_N/1
  Subtract/1 -> sum/1
  Subtract2/1 -> Abs/1
  Signal Sample and Hold2/1 -> Subtract1/2  "init0"
  " "/1 -> drawWire_m2/1
  Discrete Derivative/1 -> Bus Creator1/2, linearPower1/1  "drawWire_mpers"
  Subtract1/1 -> sum/2
  preTension_N/1 -> Terminator2/1  "preTension"
  linearPower/1 -> Bus Creator1/4  "linearPower_W"
  Bus Creator1/1 -> [linearMotion]  "linearMotion"
  [LCbot] -> Subtract2/2, Signal Sample and Hold2/1, Subtract1/1
  linearPower1/1 -> linearPower/1
  Signal Sample and Hold1/1 -> Subtract/2  "init1"
  NOT/1 -> Delay/1
  Signal Sample and Hold/1 -> " "/2  "initTest"
  [LCtop] -> Subtract2/1, Subtract/1, Signal Sample and Hold1/1
  pos_cnts/1 -> ELMO/1  "pos_counts"
  [LCtopRaw] -> Terminator6/1  "LCtop_counts"
  [LCbotRaw] -> Terminator7/1  "LCbot_counts"
  [LCTopMass] -> Bus Creator/1
  [LCBotMass] -> Bus Creator/2
  Position actual value/1 -> Subtract5/2
  Subtract3/1 -> zero start/1(pos_drv_rad)  "pos_cn"
  Velocity/1 -> vel_radpers/1
  zero start/1(pos_rad_raw) -> cntsToRad/1  "pos_cn"
  [drawWireCounts] -> Bus Creator/6  "drawWire_counts"
  cal slope/1 -> cal offset/1
  [opState] -> NOT/1
  Delay/1 -> Signal Sample and Hold/2, Signal Sample and Hold1/2, Signal Sample and Hold2/2
  Constant2/1 -> motorForce_N/2
  motorForce_N/1 -> motorForce_filt_N/1
  motorForce_filt_N/1 -> Terminator3/1
  torque_filt_Nm/1 -> Terminator4/1
  Zero Offset/1 -> Subtract5/1
  drawWire_m/1 -> Switch/1
  Zero offset in lab/1 -> Subtract6/1
  Zero offset in tank/1 -> drawWire_m/1
  cal offset/1 -> drawWire/1
  drawWire/1 -> Subtract6/2
  Subtract6/1 -> drawWire_m/2
  Switch/1 -> [drawWire]

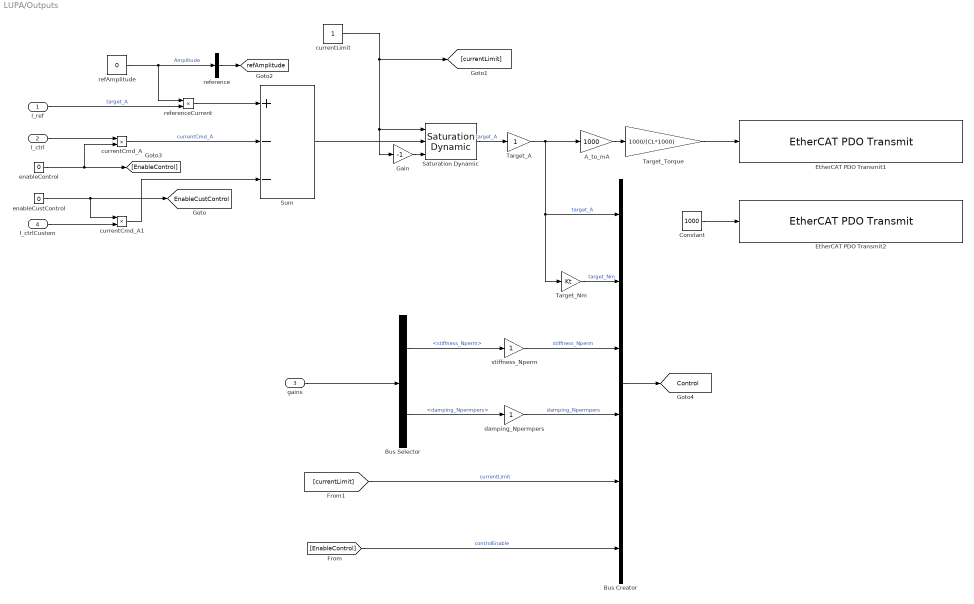
== system LUPA/Outputs ==
  I_ref : Inport
  I_ctrl : Inport  Port=2
  gains : Inport  Port=3
  I_ctrlCustom : Inport  Port=4
  A_to_mA : Gain  Gain=1000
  Bus Creator : BusCreator  Inputs=6
  Bus Selector : BusSelector  OutputSignals=stiffness_Nperm,damping_Npermpers
  Constant : Constant  Value=1000  OutDataTypeStr=uint16
  EtherCAT PDO Transmit1 : slrealtimeethercatlib/EtherCAT PDO Transmit  Priority=3  sig_name=Drive 8 (Elmo Drive ).Outputs_2.Target Torque  sig_offset=1816  sig_type=int16  type_size=16  sig_dim=1  device_id=0  sample_time=0.001000
  EtherCAT PDO Transmit2 : slrealtimeethercatlib/EtherCAT PDO Transmit  Priority=3  sig_name=Drive 8 (Elmo Drive ).Outputs_3.Max. Torque  sig_offset=1832  sig_type=uint16  type_size=16  sig_dim=1  device_id=0  sample_time=0.001000
  Gain : Gain  Gain=-1
  Saturation Dynamic : simulink/Discontinuities/Saturation Dynamic  OutMin=[]  OutMax=[]  OutDataTypeStr=Inherit: Same as second input  OutDataType=fixdt(1, 16)  OutScaling=2^-10  DoSatur=off
  Sum : Sum  Inputs=+--
  Target_A : Gain
  Target_Nm : Gain  Gain=Kt
  Target_Torque : Gain  Gain=1000/(CL*1000)  OutDataTypeStr=int16
  currentCmd_A : Product
  currentCmd_A1 : Product
  currentLimit : Constant
  damping_Npermpers : Gain
  enableControl : Constant  Value=0
  enableCustControl : Constant  Value=0
  refAmplitude : Constant  Value=0
  reference : BusCreator  Inputs=1
  referenceCurrent : Product
  stiffness_Nperm : Gain
  tag scope: Control=global, EnableCustControl=global, refAmplitude=global
  wires:
  Target_Torque/1 -> EtherCAT PDO Transmit1/1
  currentCmd_A/1 -> Sum/2  "currentCmd_A"
  currentLimit/1 -> Saturation Dynamic/1, Gain/1, [currentLimit]
  enableControl/1 -> [EnableControl], currentCmd_A/2
  I_ctrl/1 -> currentCmd_A/1
  Gain/1 -> Saturation Dynamic/3
  Saturation Dynamic/1 -> Target_A/1  "target_A"
  Bus Selector/2 -> damping_Npermpers/1  "<damping_Npermpers>"
  Target_Nm/1 -> Bus Creator/2  "target_Nm"
  Bus Selector/1 -> stiffness_Nperm/1  "<stiffness_Nperm>"
  stiffness_Nperm/1 -> Bus Creator/3  "stiffness_Nperm"
  Bus Creator/1 -> [Control]
  damping_Npermpers/1 -> Bus Creator/4  "damping_Npermpers"
  gains/1 -> Bus Selector/1
  currentCmd_A1/1 -> Sum/3
  I_ctrlCustom/1 -> currentCmd_A1/2
  enableCustControl/1 -> [EnableCustControl], currentCmd_A1/1
  [currentLimit] -> Bus Creator/5  "currentLimit"
  Sum/1 -> Saturation Dynamic/2
  I_ref/1 -> referenceCurrent/2  "target_A"
  Target_A/1 -> A_to_mA/1, Target_Nm/1, Bus Creator/1  "target_A"
  referenceCurrent/1 -> Sum/1
  refAmplitude/1 -> reference/1, referenceCurrent/1  "Amplitude"
  reference/1 -> [refAmplitude]
  [EnableControl] -> Bus Creator/6  "controlEnable"
  A_to_mA/1 -> Target_Torque/1
  Constant/1 -> EtherCAT PDO Transmit2/1

== system LUPA/Ramps ==
  EnableRamps : Constant  Value=0  OutDataTypeStr=double
  Rate Limiter : RateLimiter  RisingSlewLimit=1/rampTime  FallingSlewLimit=-1/rampTime  SampleTimeMode=inherited
  Terminator : Terminator
  wires:
  EnableRamps/1 -> Rate Limiter/1
  Rate Limiter/1 -> Terminator/1

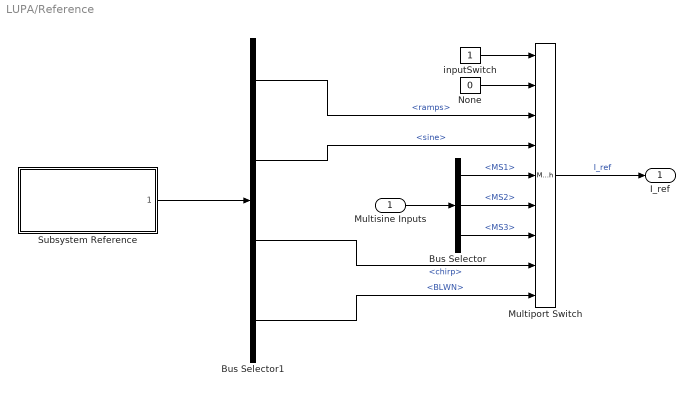
== system LUPA/Reference ==
  Multisine Inputs : Inport
  Bus Selector : BusSelector  OutputSignals=MS1,MS2,MS3
  Bus Selector1 : BusSelector  OutputSignals=ramps,sine,chirp,BLWN
  Multiport Switch : MultiPortSwitch  Inputs=8  SaturateOnIntegerOverflow=off  InputSameDT=off
  None : Constant  Value=0
  Subsystem Reference : Subsystem  ReferencedSubsystem=referenceSigs
  inputSwitch : Constant
  I_ref : Outport
  wires:
  inputSwitch/1 -> Multiport Switch/1
  Bus Selector/3 -> Multiport Switch/7  "<MS3>"
  Subsystem Reference/1 -> Bus Selector1/1
  Bus Selector/2 -> Multiport Switch/6  "<MS2>"
  Bus Selector1/2 -> Multiport Switch/4  "<sine>"
  Bus Selector1/4 -> Multiport Switch/9  "<BLWN>"
  Bus Selector1/3 -> Multiport Switch/8  "<chirp>"
  None/1 -> Multiport Switch/2
  Bus Selector/1 -> Multiport Switch/5  "<MS1>"
  Bus Selector1/1 -> Multiport Switch/3  "<ramps>"
  Multiport Switch/1 -> I_ref/1  "I_ref"
  Multisine Inputs/1 -> Bus Selector/1

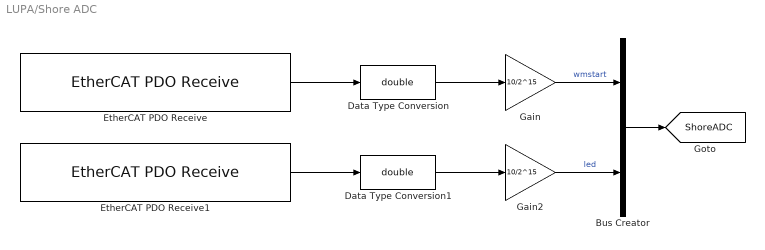
== system LUPA/Shore ADC ==
  Bus Creator : BusCreator  Inputs=2
  Data Type Conversion : DataTypeConversion  OutDataTypeStr=double  SaturateOnIntegerOverflow=off  RndMeth=Floor
  Data Type Conversion1 : DataTypeConversion  OutDataTypeStr=double  SaturateOnIntegerOverflow=off  RndMeth=Floor
  EtherCAT PDO Receive : slrealtimeethercatlib/EtherCAT PDO Receive  Priority=2  sig_name=Term 2 (EL3104).AI Standard Channel 1.Value  sig_offset=584  sig_type=int16  type_size=16  sig_dim=1  device_id=0  sample_time=0.001000
  EtherCAT PDO Receive1 : slrealtimeethercatlib/EtherCAT PDO Receive  Priority=2  sig_name=Term 2 (EL3104).AI Standard Channel 2.Value  sig_offset=616  sig_type=int16  type_size=16  sig_dim=1  device_id=0  sample_time=0.001000
  Gain : Gain  Gain=10/2^15
  Gain2 : Gain  Gain=10/2^15
  tag scope: ShoreADC=global
  wires:
  EtherCAT PDO Receive/1 -> Data Type Conversion/1
  EtherCAT PDO Receive1/1 -> Data Type Conversion1/1
  Bus Creator/1 -> [ShoreADC]
  Data Type Conversion/1 -> Gain/1
  Data Type Conversion1/1 -> Gain2/1
  Gain/1 -> Bus Creator/1  "wmstart"
  Gain2/1 -> Bus Creator/2  "led"

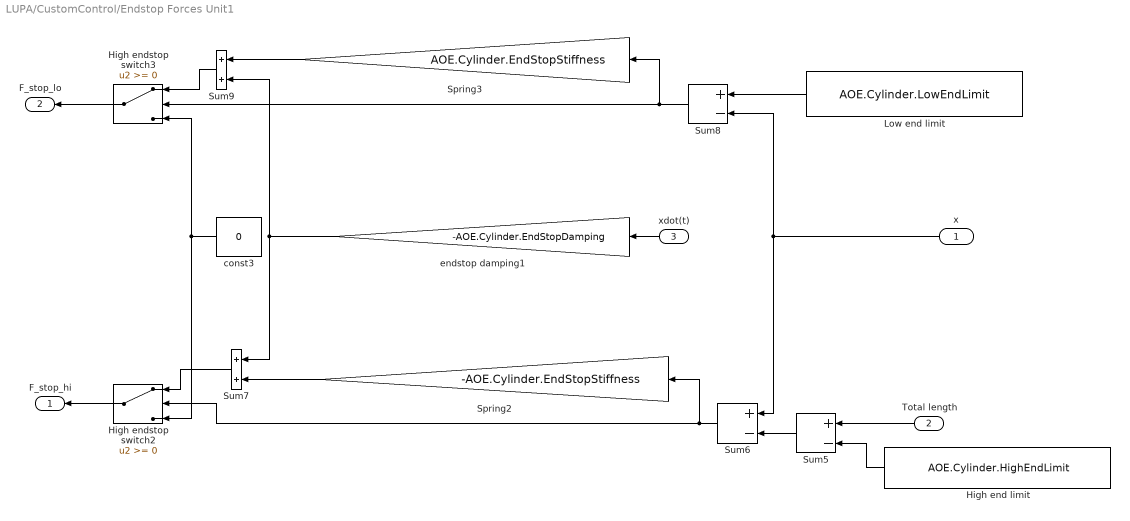
== system LUPA/CustomControl/Endstop Forces Unit1 ==
  x : Inport  OutDataTypeStr=double
  Total length : Inport  Port=2
  xdot(t) : Inport  Port=3
  High end limit : Constant  Value=AOE.Cylinder.HighEndLimit
  High endstop switch2 : Switch  SaturateOnIntegerOverflow=off  InputSameDT=off
  High endstop switch3 : Switch  SaturateOnIntegerOverflow=off  InputSameDT=off
  Low end limit : Constant  Value=AOE.Cylinder.LowEndLimit
  Spring2 : Gain  Gain=-AOE.Cylinder.EndStopStiffness
  Spring3 : Gain  Gain=AOE.Cylinder.EndStopStiffness
  Sum5 : Sum  Inputs=+-
  Sum6 : Sum  Inputs=+-
  Sum7 : Sum
  Sum8 : Sum  Inputs=+-
  Sum9 : Sum
  const3 : Constant  Value=0
  endstop damping1 : Gain  Gain=-AOE.Cylinder.EndStopDamping
  F_stop_hi : Outport  OutDataTypeStr=double
  F_stop_lo : Outport  Port=2  OutDataTypeStr=double
  wires:
  Total length/1 -> Sum5/1
  High end limit/1 -> Sum5/2
  Sum5/1 -> Sum6/2
  Sum6/1 -> High endstop switch2/2, Spring2/1
  Spring2/1 -> Sum7/2
  const3/1 -> High endstop switch3/3, High endstop switch2/3
  High endstop switch2/1 -> F_stop_hi/1
  xdot(t)/1 -> endstop damping1/1
  endstop damping1/1 -> Sum9/2, Sum7/1
  Sum7/1 -> High endstop switch2/1
  Low end limit/1 -> Sum8/1
  Sum8/1 -> High endstop switch3/2, Spring3/1
  Spring3/1 -> Sum9/1
  Sum9/1 -> High endstop switch3/1
  High endstop switch3/1 -> F_stop_lo/1
  x/1 -> Sum8/2, Sum6/1

== system LUPA/CustomControl/ForceToCurrent ==
  Force_N : Inport
  Divide : Product  Inputs=*/
  Product : Product
  Out1 : Outport
  wires:
  [sprocketPitchRadius] -> Product/2
  Product/1 -> Divide/1  "torque_Nm"
  Divide/1 -> Out1/1
  Force_N/1 -> Product/1
  [Kt] -> Divide/2

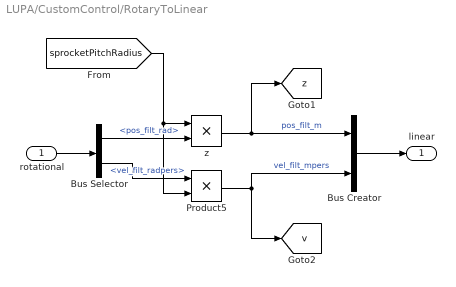
== system LUPA/CustomControl/RotaryToLinear ==
  rotational : Inport
  Bus Creator : BusCreator  Inputs=2
  Bus Selector : BusSelector  OutputSignals=pos_filt_rad,vel_filt_radpers
  Product5 : Product
  z : Product
  linear : Outport
  tag scope: v=global, z=global
  wires:
  Product5/1 -> Bus Creator/2, [v]  "vel_filt_mpers"
  Bus Selector/1 -> z/2  "<pos_filt_rad>"
  Bus Creator/1 -> linear/1
  rotational/1 -> Bus Selector/1
  z/1 -> Bus Creator/1, [z]  "pos_filt_m"
  [sprocketPitchRadius] -> Product5/2, z/1
  Bus Selector/2 -> Product5/1  "<vel_filt_radpers>"

== system LUPA/Initialization/Enabled Subsystem ==
  Enable : EnablePort
  Delay : Delay  DelayLength=1/Ts
  One : Constant  OutDataTypeStr=Inherit: Inherit via back propagation
  One1 : Constant  Value=-1  OutDataTypeStr=Inherit: Inherit via back propagation
  Sum : Sum  Inputs=|++
  Out1 : Outport
  wires:
  Sum/1 -> Out1/1
  One/1 -> Sum/1
  One1/1 -> Delay/1
  Delay/1 -> Sum/2

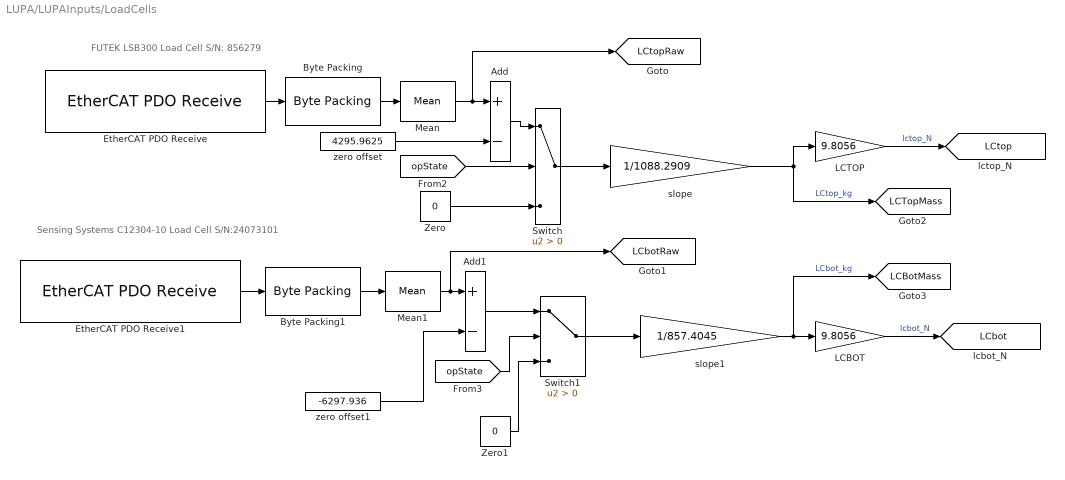
== system LUPA/LUPAInputs/LoadCells ==
  note: FUTEK LSB300 Load Cell S/N: 856279
  note: Sensing Systems C12304-10 Load Cell S/N:24073101
  Add : Sum  Inputs=+-
  Add1 : Sum  Inputs=+-
  Byte Packing : slrealtimeutilitieslib/Byte Packing  MaskPackedDataType=int32  MaskUnpackedDataTypes={'uint8'}  MaskAlignment=1
  Byte Packing1 : slrealtimeutilitieslib/Byte Packing  MaskPackedDataType=int32  MaskUnpackedDataTypes={'uint8'}  MaskAlignment=1
  EtherCAT PDO Receive : slrealtimeethercatlib/EtherCAT PDO Receive  Priority=2  sig_name=Term 6 (EL3751).PAI Samples 10.Samples  sig_offset=1240  sig_type=uint8  type_size=8  sig_dim=40  device_id=0  sample_time=0.001000
  EtherCAT PDO Receive1 : slrealtimeethercatlib/EtherCAT PDO Receive  Priority=2  sig_name=Term 5 (EL3751).PAI Samples 10.Samples  sig_offset=824  sig_type=uint8  type_size=8  sig_dim=40  device_id=0  sample_time=0.001000
  LCBOT : Gain  Gain=9.8056
  LCTOP : Gain  Gain=9.8056
  Mean : dspstat3/Mean  run=off  InputProcessing=Columns as channels (frame based)  reset_popup=None  directionMode=Each column  dimension=1  roiEnable=off  roiType=Rectangles  roiPortion=Entire ROI  roiOutput=Individual statistics for each ROI  roiFlag=off  roundingMode=Floor  overflowMode=off  outputDataTypeStr=Inherit: Same as accumulator  outputMin=[]  outputMax=[]  outputLastDataTypeStr=Inherit: Same as accumulator
  Mean1 : dspstat3/Mean  run=off  InputProcessing=Columns as channels (frame based)  reset_popup=None  directionMode=Each column  dimension=1  roiEnable=off  roiType=Rectangles  roiPortion=Entire ROI  roiOutput=Individual statistics for each ROI  roiFlag=off  roundingMode=Floor  overflowMode=off  outputDataTypeStr=Inherit: Same as accumulator  outputMin=[]  outputMax=[]  outputLastDataTypeStr=Inherit: Same as accumulator
  Switch : Switch  Criteria=u2 > Threshold  SaturateOnIntegerOverflow=off  InputSameDT=off
  Switch1 : Switch  Criteria=u2 > Threshold  SaturateOnIntegerOverflow=off  InputSameDT=off
  Zero : Constant  Value=0  OutDataTypeStr=Inherit: Inherit via back propagation
  Zero1 : Constant  Value=0  OutDataTypeStr=Inherit: Inherit via back propagation
  slope : Gain  Gain=1/1088.2909
  slope1 : Gain  Gain=1/857.4045
  zero offset : Constant  Value=4295.9625
  zero offset1 : Constant  Value=-6297.936
  tag scope: LCBotMass=global, LCTopMass=global, LCbot=global, LCbotRaw=global, LCtop=global, LCtopRaw=global
  wires:
  Byte Packing1/1 -> Mean1/1
  EtherCAT PDO Receive1/1 -> Byte Packing1/1
  Mean1/1 -> [LCbotRaw], Add1/1
  Byte Packing/1 -> Mean/1
  Switch/1 -> slope/1
  EtherCAT PDO Receive/1 -> Byte Packing/1
  slope/1 -> LCTOP/1, [LCTopMass]  "LCtop_kg"
  LCTOP/1 -> [LCtop]  "lctop_N"
  LCBOT/1 -> [LCbot]  "lcbot_N"
  slope1/1 -> [LCBotMass], LCBOT/1  "LCbot_kg"
  Add1/1 -> Switch1/1
  zero offset1/1 -> Add1/2
  Zero/1 -> Switch/3
  [opState] -> Switch/2
  [opState] -> Switch1/2
  Zero1/1 -> Switch1/3
  Switch1/1 -> slope1/1
  Mean/1 -> [LCtopRaw], Add/1
  Add/1 -> Switch/1
  zero offset/1 -> Add/2

== system LUPA/LUPAInputs/zero start ==
  pos_drv_rad : Inport
  Switch : Switch  Criteria=u2 > Threshold  SaturateOnIntegerOverflow=off  InputSameDT=off
  Zero : Constant  Value=0  OutDataTypeStr=double
  pos_rad_raw : Outport
  wires:
  [opState] -> Switch/2
  Switch/1 -> pos_rad_raw/1
  pos_drv_rad/1 -> Switch/1
  Zero/1 -> Switch/3

== matlab function LUPA/CustomControl/Temperature Chamber1 Box Unit1 ==
  data: P input; T output; Rs input; V input; m input
function T = fcn(P,Rs,V,m)
T = P*V/(m*Rs);

== matlab function LUPA/CustomControl/Temperature Chamber2 Box Unit1 ==
  data: P input; T output; Rs input; V input; m input
function T = fcn(P,Rs,V,m)

T = P*V/(m*Rs);
